simulink model "EnvelopeDetection-1"  (R2019b)
settings: Solver=VariableStepAuto  StartTime=0.0  StopTime=0.05  RelTol=1e-3
settings Model: Creator=au192593  LastModifiedBy=au192593

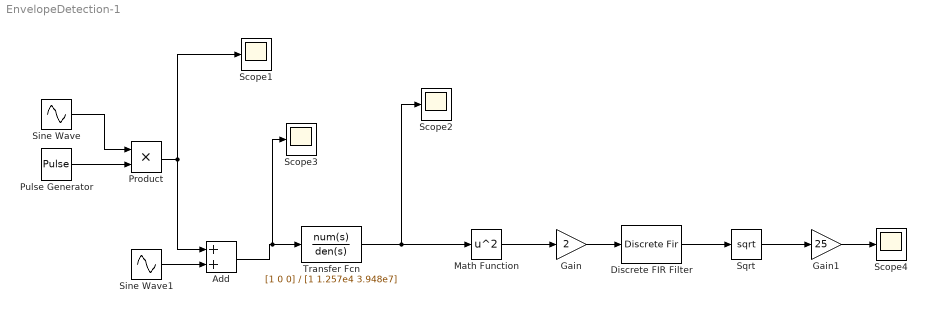
== system EnvelopeDetection-1 ==
  Add : Sum
  Discrete FIR Filter : DiscreteFir  Coefficients=1/1000.*ones(1, 1000)  SampleTime=2e-7
  Gain : Gain  Gain=2
  Gain1 : Gain  Gain=25
  Math Function : Math  Operator=square  SignedPower=off  SaturateOnIntegerOverflow=on
  Product : Product
  Pulse Generator : DiscretePulseGenerator  PulseType=Time based  Period=1/100  PulseWidth=20
  Scope{1..4} (4 alike) : Scope
  Sine Wave : Sin  Amplitude=0.2  Frequency=7.53e5  SampleTime=0
  Sine Wave1 : Sin  Frequency=314.1593  SampleTime=0
  Sqrt : Sqrt  SaturateOnIntegerOverflow=on
  Transfer Fcn : TransferFcn  Numerator=[1 0 0]  Denominator=[1 1.257e4 3.948e7]
  wires:
  Math Function/1 -> Gain/1
  Gain/1 -> Discrete FIR Filter/1
  Discrete FIR Filter/1 -> Sqrt/1
  Sine Wave/1 -> Product/1
  Product/1 -> Add/1, Scope1/1
  Pulse Generator/1 -> Product/2
  Sine Wave1/1 -> Add/2
  Add/1 -> Scope3/1, Transfer Fcn/1
  Transfer Fcn/1 -> Scope2/1, Math Function/1
  Sqrt/1 -> Gain1/1
  Gain1/1 -> Scope4/1
